simulink model "Lokomat_Simulation"  (R2022b)
settings: Solver=FixedStepAuto  StartTime=0.0  StopTime=4  FixedStep=0.001  RelTol=1e-3
values from neighbouring files (symbols this model uses):
  kd = max(kd_hip)    [RMSE_code.m]    (also in Step_Hip.m = kd; Step_Knee.m = kd; Step_Response.m = max(kd_vec))
  kp = max(RMSE{length(kd_hip)}(:,1))    [RMSE_code.m]    (also in RMSE_hip.m = kp_vec_use(j); RMSE_knee.m = kp_vec_use(j); Step_Hip.m = kp; Step_Knee.m = kp)
undefined symbols (not defined in the file or in its folder): X, Y, Z
libraries: sm_lib x82, nesl_utility x9, simulink x6
(part 3 of 3)

== matlab function Lokomat_Simulation/Predetermined trajectory ==
  data: x input; Desired_Hip_Fl output; Desired_Hip_Ab output; Desierd_Knee_Fl output

function [Desired_Hip_Fl,Desired_Hip_Ab,Desierd_Knee_Fl] = desired_trajectory(x)
x=x-floor(x);
 a0 =     -0.3548; 
       a1 =       0.02918;  
       b1 =     0.3386;  
       a2 =      0.2412;  
       b2 =      -0.141;  
       a3 =     0.001263;  
       b3 =     -0.07783;  
       a4 =     0.01228;  
       b4 =    -0.008624;  
       a5 =   0.006195;  
       b5 =      -0.01385;  
       a6 =   -0.003767;  
       b6 =   -0.002801; 
       w =       6.292; 

Desierd_Knee_Fl = ( a0 + a1*cos(x*w) + b1*sin(x*w) +  a2*cos(2*x*w) + b2*sin(2*x*w) + a3*cos(3*x*w) + b3*sin(3*x*w) + a4*cos(4*x*w) + b4*sin(4*x*w) + a5*cos(5*x*w) + b5*sin(5*x*w) + a6*cos(6*x*w) + b6*sin(6*x*w));
a0 =     0.1298 ;
       a1 =       0.3635      ;
       b1 =     -0.04958 ;
       a2 =      -0.0579  ;
       b2 =    -0.02446 ;
       a3 =     -0.002222  ;
       b3 =   0.02576  ;
       a4 =   -0.001088  ;
       b4 =     -0.002438 ;
       a5 =    -0.003805  ;
       b5 =    0.002449 ;
       w =       6.377;


Desired_Hip_Fl = a0 + a1*cos(x*w) + b1*sin(x*w) +  a2*cos(2*x*w) + b2*sin(2*x*w) + a3*cos(3*x*w) + b3*sin(3*x*w) + a4*cos(4*x*w) + b4*sin(4*x*w) + a5*cos(5*x*w) + b5*sin(5*x*w);

a1 =       5.514;
b1 =       5.793;
c1 =      0.4861;
a2 =       3.071;
b2 =       2.574;
c2 =     -0.3713;
a3 =       1.085;
b3 =       19.73;
c3 =      -1.814;
a4 =      0.8685;
b4 =       14.16;
c4 =       1.821;
a5 =      0.2569;
b5 =       31.41;
c5 =      -2.433;

Desired_Hip_Ab=(a1*sin(b1*x+c1) + a2*sin(b2*x+c2) + a3*sin(b3*x+c3) + a4*sin(b4*x+c4) + a5*sin(b5*x+c5))*pi/180;

== matlab function Lokomat_Simulation/Controller  ==
  data: Par input; Knee_Flex input; Int_Pris input; Ext_Pris input; Desired_Knee_Flex input; Desired_Int input; Desired_Ext input; Trq_Knee output; Force_Int output; Force_Ext output; dKnee input; dInt input; dExt input
function [Trq_Knee,Force_Int,Force_Ext] = fcn(Par, Knee_Flex,Int_Pris,Ext_Pris,Desired_Knee_Flex,Desired_Int, Desired_Ext, dKnee, dInt, dExt)
%% Knee Controller
% The amount of desired torque should be determinded by knowing the amount
% of desired and actual trajectory of knee.

%question regarding kp increase 
%kv = 0.5
%kp1 = 20
%kp2 = 700
%kp3 = 148300
%kp4 = 148500
%kv2 = 
kp =Par(1);
kv =Par(2); 

theta_des = Desired_Knee_Flex;
theta_act = Knee_Flex;
theta_diff = theta_des-theta_act;
dtheta_act = dKnee(1);
dtheta_des = dKnee(2);
dtheta_diff = dtheta_des-dtheta_act;

out = kp*(theta_diff)+kv*(dtheta_diff);

Trq_Knee= out;

%% Hip Controller
% In order to control the flexion/extension and abduction/adduction of hip,
% the amount of forces for internal and external actuators should be
% determinded as the desired and actual trajectory of hip are available and
% also the inverse kinematic can map them to prismatic joint space.


kp_int = Par(1);
kv_int = Par(2);

int_des = Desired_Int;
int_act = Int_Pris;
int_diff = int_des-int_act;
dint_act = dInt(1);
dint_des = dInt(2);
dint_diff = dint_des-dint_act;


out_int =kp_int*(int_diff)+kv_int*(dint_diff);

kp_ext= kp_int;
kv_ext = kv_int;

ext_des = Desired_Ext;
ext_act = Ext_Pris;
ext_diff = ext_des-ext_act;
dExt_act = dExt(1);
dExt_des = dExt(2);
dExt_diff = dExt_des-dExt_act;

out_ext = kp_ext*(ext_diff)+kv_ext*(dExt_diff);


Force_Int=out_int;
Force_Ext=out_ext;

== matlab function Lokomat_Simulation/Inverse Kinematic  ==
  data: Hip_Flex input; Hip_Abd input; Pris_int output; Pris_ext output

function [Pris_int,Pris_ext] = fcn(Hip_Flex,Hip_Abd)

%% Data of Pelvis Plate
RR=eye(3);
F=.2; % frontal distance between fixed plate and pelvis plate
T=0; % transverse distance between fixed plate and pelvis plate
L=0; % lateral distance between fixed plate and pelvis plate
%%data of thigh bar with back shaft to revolute joint

m=.34; % distance of center of back shaft of thigh with hip joint which it is determinded for diiferent patients with different length of their thighs (34cm) 
n=.105+.0175; % distance of back plate of thigh bar to revolute joint which is fixed
% r=sqrt(m^2+n^2); %radius of revolute joint relative to hip joint
% phi=atan(n/m); % angular position of revolute joint relative to thigh bar
r=[0 -1 0;1 0 0;0 0 1];
ri=[0 1 0;-1 0 0;0 0 1];
vc=[-n,0,-m]';
vc=r*vc;

d=[.1105 -.208 -.098]'; % distance between pelvis plate and hip joint
of=[.31 .1805 .467]'; % distance from revolute joint of hip actuators to fixed plate
R = [1 0 0; 0 cos(Hip_Abd) -sin(Hip_Abd); 0 sin(Hip_Abd) cos(Hip_Abd)]*[cos(Hip_Flex) 0 sin(Hip_Flex); 0 1 0; -sin(Hip_Flex) 0 cos(Hip_Flex)]; % rotation matrix of hip respect to pelvis


vc_R=R*vc;
vc_RR=RR*(ri*vc_R+d);
%% data of parallel mechanism for hip actuators
q=.18; %length of right bars of parallel mechanism of hip actuator
l=.26; %length of left bar of parallel mechanism of hip actuator


%%Lateral movemnt of frontal plate of actuators

Dy=vc_RR(2)+L+of(2);
Dx=vc_RR(1)+F+of(1);
Dz=vc_RR(3)+T+of(3);
C=.205; % distance between two axis of prismatic hip actuators
thetaq=acos((Dy+C/2)/q); %angle of right bars of parallel mechanism of hip actuator
thetal=acos((-Dy+C/2)/l); %angle of left bar of parallel mechanism of hip actuator
% Th=atan(Dz/Dx); % angle of hip actuators respect to horizon
Se=sqrt(Dx^2+Dz^2);
Si=Se;
dc=.165; % offsets
Pris_ext=Se-(dc+q*sin(thetaq)); % the amount of traveling external prismatic actuator
Pris_int=Si-(dc+l*sin(thetal)); % the amount of traveling internal prismatic actuator
